simulink model "tbursting_linear"  (R2015a)
settings: Solver=ode45  StartTime=0.0  StopTime=10.0  RelTol=1e-3
values from neighbouring files (symbols this model uses):
  alpha_const = 0.0    (= 0)    [averagedRelayOutput.m]    (also in bursting_linearised.m = 0.1; fastSlow.m; manParamsNullclines.m; manipulateParameters.m = getappdata(hObject.Parent,'alpha_const'))
  beta = 0.37    [averagedRelayOutput.m]    (also in bursting_linearised.m = 0.27; compareApproximations.m = 1.5; fastSlow.m; fast_nullcline_winged_cusp.m = 0.5)
  fast_plant_X0 = -1.0    (= -1)    [averagedRelayOutput.m]    (also in bursting_linearised.m = -1.05; fastSlow.m; fast_nullcline_winged_cusp.m; hRose.m = 0)
  gamma = 0    [averagedRelayOutput.m]    (also in bursting_linearised.m = 1; compareApproximations.m = 1; fastSlow.m; fast_nullcline_winged_cusp.m = 1)
  slow_plant_X0 = -1.0    (= -1)    [averagedRelayOutput.m]    (also in bursting_linearised.m = -1.05; fastSlow.m; fast_nullcline_winged_cusp.m = -2; hRose.m = -10)
  ts = 1    [averagedRelayOutput.m]    (also in bursting_linearised.m; compareApproximations.m; fastSlow.m; fast_nullcline_winged_cusp.m)
  tus = 800    [averagedRelayOutput.m]    (also in bursting_linearised.m; fastSlow.m; manParamsNullclines.m; manipulateParameters.m = getappdata(hObject.Parent,'tus'))
  ultra_slow_plant_X0 = 0.45    [averagedRelayOutput.m]    (also in bursting_linearised.m = 0; fastSlow.m; hRose.m = 2000; manParamsNullclines.m)
settings Model: Creator=ra428  LastModifiedBy=ra428

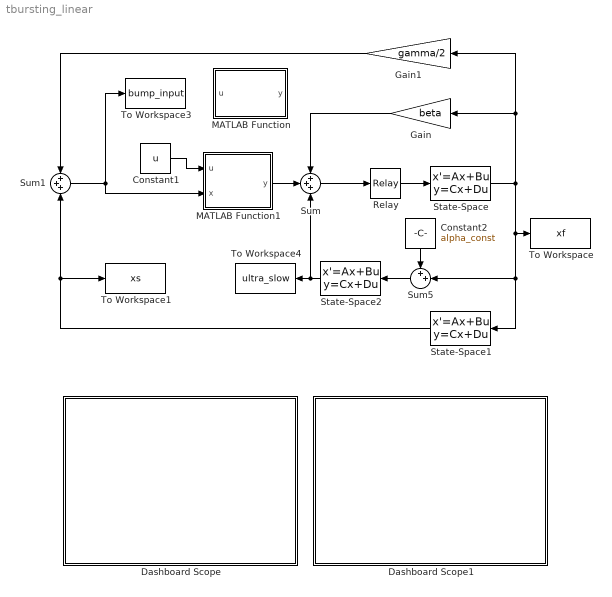
== system tbursting_linear ==
  Constant1 : Constant  Value=u
  Constant2 : Constant  Value=alpha_const
  Dashboard Scope : Subsystem  DialogController=hmiCreateDDGDialog  IsWebBlock=on  mask(MathWorksWebBlock){webBlockId=d46ec359-3d6b-4022-9ce1-54e1038fb040, webBlockType=sdiscope, ShowInitialText=on, HMISrcModelName=untitled}
      mask prompts: webBlockId "WebBlock Id"; webBlockType "WebBlock Type"; HMISrcModelName "Source Model"
      mask Help: helpview([docroot '/mapfiles/simulink.map'], 'hmi_scope')
      mask Display:
      | if strcmp(get_param(bdroot(gcb),'BlockDiagramType'), 'library')
      |     image([(matlabroot) '/toolbox/simulink/hmi/icons/DashboardScope.png']);
      | end
  Dashboard Scope1 : Subsystem  DialogController=hmiCreateDDGDialog  IsWebBlock=on  mask(MathWorksWebBlock){webBlockId=b7f05316-8e8a-4393-b217-3b7ed9d7156b, webBlockType=sdiscope, ShowInitialText=on, HMISrcModelName=untitled}
      mask prompts: webBlockId "WebBlock Id"; webBlockType "WebBlock Type"; HMISrcModelName "Source Model"
      mask Help: helpview([docroot '/mapfiles/simulink.map'], 'hmi_scope')
      mask Display:
      | if strcmp(get_param(bdroot(gcb),'BlockDiagramType'), 'library')
      |     image([(matlabroot) '/toolbox/simulink/hmi/icons/DashboardScope.png']);
      | end
  Gain : Gain  Gain=beta
  Gain1 : Gain  Gain=gamma/2
  MATLAB Function : MATLAB Function  TreatAsAtomicUnit=on
  MATLAB Function1 : MATLAB Function  TreatAsAtomicUnit=on
  Relay : Relay  OffOutputValue=-1
  State-Space : StateSpace  A=-1/tf  B=1/tf  D=0  X0=fast_plant_X0
  State-Space1 : StateSpace  A=-1/ts  B=1/ts  D=0  X0=slow_plant_X0
  State-Space2 : StateSpace  A=-1/tus  B=-1/tus  D=0  X0=ultra_slow_plant_X0
  Sum : Sum  Inputs=+++
  Sum1 : Sum  Inputs=+++
  Sum5 : Sum  Inputs=++|
  To Workspace : ToWorkspace  VariableName=xf  SaveFormat=Timeseries  SampleTime=-1
  To Workspace1 : ToWorkspace  VariableName=xs  SaveFormat=Timeseries  SampleTime=-1
  To Workspace3 : ToWorkspace  VariableName=bump_input  SaveFormat=Timeseries  SampleTime=-1
  To Workspace4 : ToWorkspace  VariableName=ultra_slow  SaveFormat=Timeseries  SampleTime=-1
  wires:
  Sum/1 -> Relay/1
  Sum1/1 -> To Workspace3/1, MATLAB Function1/2(x)
  Gain/1 -> Sum/1
  Gain1/1 -> Sum1/1
  Relay/1 -> State-Space/1
  State-Space/1 -> State-Space1/1, Sum5/2, To Workspace/1, Gain/1, Gain1/1
  State-Space1/1 -> Sum1/3, To Workspace1/1
  Constant2/1 -> Sum5/1
  Sum5/1 -> State-Space2/1
  State-Space2/1 -> Sum/3, To Workspace4/1
  Constant1/1 -> MATLAB Function1/1(u)
  MATLAB Function1/1(y) -> Sum/2

== system tbursting_linear/Dashboard Scope ==

== system tbursting_linear/Dashboard Scope1 ==

== matlab function tbursting_linear/MATLAB Function1 ==
  data: u input; x input; y output
function y = fcn(u,x)
%#codegen
if (x < -2-u)
    y = -2;
elseif (x > 2-u)
    y = -2;
elseif and( x>=-2-u,x < -u)
    y = (x+u);
else
    y = -(x+u);
end

== matlab function tbursting_linear/MATLAB Function ==
  data: u input; y output
function y = fcn(u)
%#codegen
if (u < -2)
    y = -1;
elseif (u > 2)
    y = -1;
elseif and( u>=-2,u < 0)
    y = 0.5*u;
else
    y = -0.5*u;
end
